simulink model "PUMA_8MM"  (Simulink 8.6)
settings: Solver=ode5  StartTime=0.0  StopTime=3  FixedStep=0.003  RelTol=1e-3
undefined symbols (not defined in the file): magnitude
libraries: vrlib x8, simulink x5
(part 1 of 2)
settings Model: Creator=Igor  LastModifiedBy=User
settings OptimizationCC: InitFltsAndDblsToZero=on
settings DebuggingCC: FcnCallInpInsideContextMsg=UseLocalSettings
settings SFSimCC: SimParseCustomCode=off

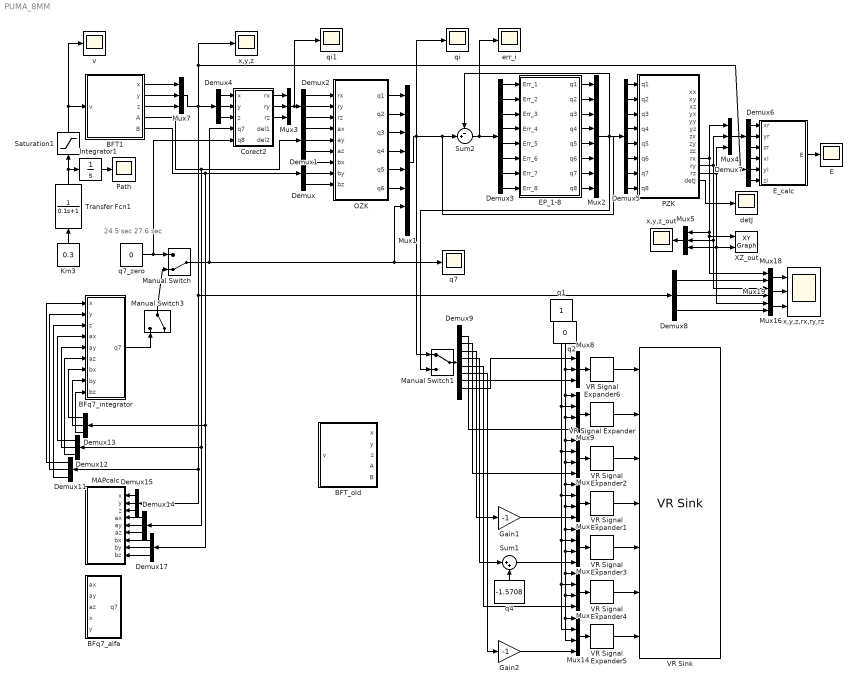
== system PUMA_8MM ==
  note: 24.5 sec
      | 27.6 sec
  BFT1 : Subsystem
  BFT_old : Subsystem
  BFq7_alfa : MATLAB Function  TreatAsAtomicUnit=on
  BFq7_integrator : Subsystem
  Corect2 : MATLAB Function  TreatAsAtomicUnit=on
  Demux{,1..2,4,6..8,11..15,17} (13 alike) : Demux  Outputs=3
  Demux3 : Demux  Outputs=8
  Demux5 : Demux  Outputs=8
  Demux9 : Demux  Outputs=8
  E : Scope
  EP_1-8 : Subsystem
  E_calc : MATLAB Function  TreatAsAtomicUnit=on
  Gain1 : Gain  Gain=-1
  Gain2 : Gain  Gain=-1
  Integrator1 : Integrator
  Km3 : Constant  Value=0.3
  MAPcalc : Subsystem
  Manual Switch : ManualSwitch  CurrentSetting=0
  Manual Switch1 : ManualSwitch
  Manual Switch3 : ManualSwitch  CurrentSetting=0
  Mux1 : Mux  Inputs=8
  Mux{9..14} (6 alike) : Mux
  Mux16 : Mux  Inputs=2
  Mux18 : Mux  Inputs=2
  Mux19 : Mux  Inputs=2
  Mux2 : Mux  Inputs=8
  Mux{3..5,7..8} (5 alike) : Mux  Inputs=3
  OZK : MATLAB Function  TreatAsAtomicUnit=on
  PZK : MATLAB Function  TreatAsAtomicUnit=on
  Path : Scope
  Saturation1 : Saturate  UpperLimit=10  LowerLimit=0.001
  Sum1 : Sum  Inputs=|++
  Sum2 : Sum  Inputs=-+|
  Transfer Fcn1 : TransferFcn  Denominator=[0.1 1]
  VR Signal Expander{,1..5} (6 alike) : vrlib/VR Signal Expander  outwidth=4  outidx=[1 2 3 4]
  VR Signal Expander6 : vrlib/VR Signal Expander  outwidth=3  outidx=[1 2 3]
  VR Sink : vrlib/VR Sink  InstantiateOnLoad=on  SampleTime=-1  ViewEnable=on  RemoteChange=off  RemoteView=off  FieldsWritten=q7_block1.translation.3.1.1.double#q1_block3.rotation.4.1.1.double#q2_block5.rotation.4.1.1.double#q3_block7.rotation.4.1.1.double#q4_block8.rotation.4.1.1.double#q5_block10.rotation.4.1.1.double#q6_block11.rotation.4.1.1.double  WorldFileName=MM_3Dmodel.wrl  WorldDescription=MM_3Dmodel  AutoView=on  VideoDimensions=[]  AllowVariableSize=off  FigureProperties="{'Position', 'Name', 'Viewpoint', 'CameraBound', 'CameraDirection', 'CameraPosition', 'CameraUpVector', 'ZoomFactor', 'Antialiasing', 'Headlight', 'Lighting', 'NavPanel', 'Sound', 'StatusBar', 'Stereo3D', 'Stereo3DCameraOffset', 'Stereo3DHIT', 'ToolBar', 'Textures', 'Transparency', 'Triad', 'Wireframe', 'NavZones', 'NavMode', 'NavSpeed', 'CaptureFileFormat', 'CaptureFileName', 'Record2DCompressMethod', 'Record2DCompressQuality', 'Record2D', 'Record2DFileName', 'Record2DFPS'; [9.3400000000000000e+02   2.7200000000000000e+02   8.2600000000000000e+02   5.2800000000000000e+02], 'MM_3Dmodel', '', 'on', [-6.5943356188839664e-01  -2.5114047294941466e-01  -7.0857310159359332e-01], [2.3358426713746256e+00   1.1531799680057284e+00   2.3142922974527869e+00], [-1.9468492056750838e-01   9.6744405949295276e-01  -1.6170891581923202e-01], [1.0000000000000000e+00], 'on', 'on', 'on', 'halfbar', 'on', 'on', 'off', [1.0000000149011612e-01], [0.0000000000000000e+00], 'on', 'on', 'on', 'none', 'off', 'off', 'fly', 'normal', 'tif', '%f_anim_%n.tif', 'auto', [7.5000000000000000e+01], 'off', '%f_anim_%n.avi', [1.5000000000000000e+01]}"
  XZ_out : simulink/Sinks/XY Graph  xmin=-0.5  xmax=1.5  ymin=-0.5  ymax=1.5  st=-1
  detJ : Scope
  err_i : Scope
  q1 : Constant
  q2 : Constant  Value=0
  q4 : Constant  Value=-1.5708
  q7 : Scope
  q7_zero : Constant  Value=0
  qi : Scope
  qi1 : Scope
  v : Scope
  x,y,z : Scope
  x,y,z,rx,ry,rz : Scope  NumInputPorts=3
  x,y,z_out : Scope
  wires:
  E_calc/1(E) -> E/1
  Integrator1/1 -> Path/1
  Saturation1/1 -> v/1, BFT1/1(v)
  Demux/1 -> OZK/7(bx)
  Demux/2 -> OZK/8(by)
  Demux/3 -> OZK/9(bz)
  Demux1/1 -> OZK/4(ax)
  Demux1/2 -> OZK/5(ay)
  Demux1/3 -> OZK/6(az)
  Demux2/1 -> OZK/1(rx)
  Demux2/2 -> OZK/2(ry)
  Demux2/3 -> OZK/3(rz)
  Mux1/1 -> Sum2/2, Demux5/1, Manual Switch1/1, qi/1
  BFT1/3(z) -> Mux7/3
  Demux3/1 -> EP_1-8/1(Err_1)
  Demux3/2 -> EP_1-8/2(Err_2)
  Demux3/3 -> EP_1-8/3(Err_3)
  Demux3/4 -> EP_1-8/4(Err_4)
  Demux3/5 -> EP_1-8/5(Err_5)
  Demux3/6 -> EP_1-8/6(Err_6)
  EP_1-8/1(q1) -> Mux2/1
  EP_1-8/2(q2) -> Mux2/2
  EP_1-8/3(q3) -> Mux2/3
  EP_1-8/4(q4) -> Mux2/4
  EP_1-8/5(q5) -> Mux2/5
  EP_1-8/6(q6) -> Mux2/6
  Demux3/7 -> EP_1-8/7(Err_7)
  Demux3/8 -> EP_1-8/8(Err_8)
  EP_1-8/7(q7) -> Mux2/7
  EP_1-8/8(q8) -> Mux2/8
  Mux7/1 -> Demux4/1, Demux8/1, Demux11/1, Demux15/1, Demux7/1, x,y,z/1
  Demux5/1 -> PZK/1(q1)
  Demux5/2 -> PZK/2(q2)
  Demux5/3 -> PZK/3(q3)
  Demux5/4 -> PZK/4(q4)
  Demux5/5 -> PZK/5(q5)
  Demux5/6 -> PZK/6(q6)
  Demux5/7 -> PZK/7(q7)
  Demux5/8 -> PZK/8(q8)
  Demux6/1 -> E_calc/1(xr)
  Demux6/2 -> E_calc/2(yr)
  Demux6/3 -> E_calc/3(zr)
  Mux4/1 -> Demux6/1
  Demux7/1 -> E_calc/4(xi)
  Demux7/2 -> E_calc/5(yi)
  Demux7/3 -> E_calc/6(zi)
  OZK/1(q1) -> Mux1/1
  OZK/3(q3) -> Mux1/3
  OZK/2(q2) -> Mux1/2
  OZK/4(q4) -> Mux1/4
  OZK/5(q5) -> Mux1/5
  OZK/6(q6) -> Mux1/6
  Demux8/3 -> Mux16/2
  Demux8/2 -> Mux19/2
  Demux8/1 -> Mux18/2
  Mux18/1 -> x,y,z,rx,ry,rz/1
  Mux19/1 -> x,y,z,rx,ry,rz/2
  Mux16/1 -> x,y,z,rx,ry,rz/3
  PZK/10(rx) -> Mux4/1, Mux18/1, XZ_out/1, Mux5/1
  PZK/11(ry) -> Mux4/2, Mux5/2, Mux19/1
  PZK/12(rz) -> Mux4/3, Mux16/1, XZ_out/2, Mux5/3
  Mux3/1 -> qi1/1, Demux2/1
  Mux8/1 -> VR Signal Expander6/1
  q2/1 -> Mux8/2, Mux9/1, Mux9/3, Mux11/1, Mux10/1, Mux10/3, Mux12/1, Mux12/3, Mux13/1, Mux13/3, Mux14/1, Mux14/3, Mux11/3
  Mux9/1 -> VR Signal Expander/1
  q1/1 -> Mux9/2, Mux11/2, Mux10/2, Mux12/2, Mux13/2, Mux14/2
  Demux9/1 -> Mux9/4
  Demux9/7 -> Mux8/3
  Mux10/1 -> VR Signal Expander1/1
  Demux9/3 -> Gain1/1
  Mux11/1 -> VR Signal Expander2/1
  Demux9/2 -> Mux11/4
  Mux12/1 -> VR Signal Expander3/1
  Demux9/4 -> Sum1/1
  Mux13/1 -> VR Signal Expander4/1
  Demux9/5 -> Mux13/4
  Demux9/8 -> Mux8/1
  Mux14/1 -> VR Signal Expander5/1
  Gain1/1 -> Mux10/4
  Demux9/6 -> Gain2/1
  VR Signal Expander6/1 -> VR Sink/1
  VR Signal Expander/1 -> VR Sink/2
  VR Signal Expander2/1 -> VR Sink/3
  VR Signal Expander1/1 -> VR Sink/4
  VR Signal Expander3/1 -> VR Sink/5
  VR Signal Expander4/1 -> VR Sink/6
  VR Signal Expander5/1 -> VR Sink/7
  Gain2/1 -> Mux14/4
  Manual Switch1/1 -> Demux9/1
  Sum1/1 -> Mux12/4
  q4/1 -> Sum1/2
  Sum2/1 -> err_i/1, Demux3/1
  q7_zero/1 -> Manual Switch/1, Corect2/5(q8)
  BFT1/2(y) -> Mux7/2
  BFT1/1(x) -> Mux7/1
  BFT1/4(A) -> Demux12/1, Demux14/1, Demux1/1
  BFT1/5(B) -> Demux13/1, Demux17/1, Demux/1
  Mux2/1 -> Manual Switch1/2, Sum2/1
  Demux11/1 -> BFq7_integrator/1(x)
  Demux11/2 -> BFq7_integrator/2(y)
  Demux11/3 -> BFq7_integrator/3(z)
  Demux12/1 -> BFq7_integrator/4(ax)
  Demux12/2 -> BFq7_integrator/5(ay)
  Demux12/3 -> BFq7_integrator/6(az)
  Demux13/1 -> BFq7_integrator/7(bx)
  Demux13/2 -> BFq7_integrator/8(by)
  Demux13/3 -> BFq7_integrator/9(bz)
  Manual Switch3/1 -> Manual Switch/2
  BFq7_integrator/1(q7) -> Manual Switch3/1
  Km3/1 -> Transfer Fcn1/1
  Transfer Fcn1/1 -> Saturation1/1, Integrator1/1
  PZK/13(detJ) -> detJ/1
  Demux17/3 -> MAPcalc/9(bz)
  Demux17/2 -> MAPcalc/8(by)
  Demux17/1 -> MAPcalc/7(bx)
  Demux14/3 -> MAPcalc/6(az)
  Demux14/2 -> MAPcalc/5(ay)
  Demux14/1 -> MAPcalc/4(ax)
  Demux15/3 -> MAPcalc/3(z)
  Demux15/2 -> MAPcalc/2(y)
  Demux15/1 -> MAPcalc/1(x)
  Manual Switch/1 -> q7/1, Mux1/7, Corect2/4(q7)
  Corect2/1(rx) -> Mux3/1
  Corect2/2(ry) -> Mux3/2
  Corect2/3(rz) -> Mux3/3
  Demux4/1 -> Corect2/1(x)
  Demux4/2 -> Corect2/2(y)
  Demux4/3 -> Corect2/3(z)
  Mux5/1 -> x,y,z_out/1

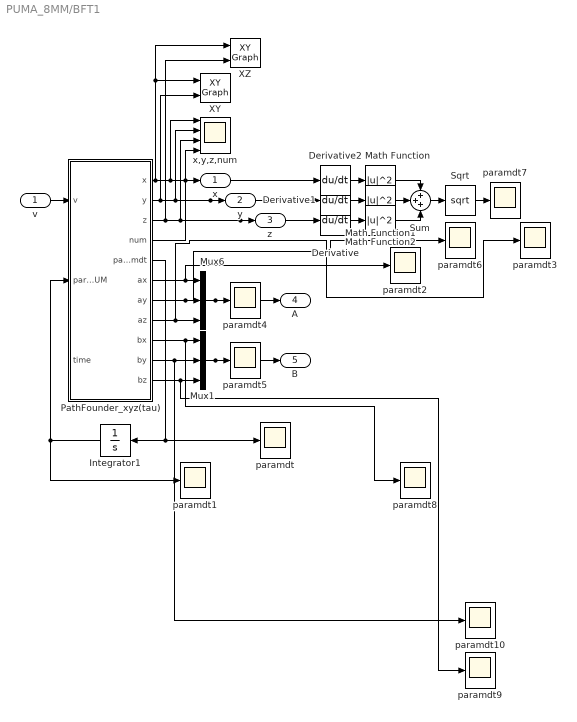
== system PUMA_8MM/BFT1 ==
  v : Inport
  Derivative : Derivative
  Derivative1 : Derivative
  Derivative2 : Derivative
  Integrator1 : Integrator
  Math Function : Math  Operator=magnitude^2  SaturateOnIntegerOverflow=on
  Math Function1 : Math  Operator=magnitude^2  SaturateOnIntegerOverflow=on
  Math Function2 : Math  Operator=magnitude^2  SaturateOnIntegerOverflow=on
  Mux1 : Mux  Inputs=3
  Mux6 : Mux  Inputs=3
  PathFounder_xyz(tau) : MATLAB Function  TreatAsAtomicUnit=on
  Sqrt : Sqrt  SaturateOnIntegerOverflow=on
  Sum : Sum  Inputs=+++
  XY : simulink/Sinks/XY Graph  xmin=-0.5  xmax=1.5  ymin=0  ymax=2  st=-1
  XZ : simulink/Sinks/XY Graph  xmin=-0.5  xmax=1.5  ymin=-0.5  ymax=1.5  st=-1
  paramdt{,1..10} (11 alike) : Scope
  x,y,z,num : Scope  NumInputPorts=4
  x : Outport
  y : Outport  Port=2
  z : Outport  Port=3
  A : Outport  Port=4
  B : Outport  Port=5
  wires:
  v/1 -> PathFounder_xyz(tau)/1(v)
  PathFounder_xyz(tau)/4(num) -> x,y,z,num/4
  PathFounder_xyz(tau)/3(z) -> XZ/2, z/1, Derivative/1, x,y,z,num/3
  PathFounder_xyz(tau)/2(y) -> y/1, Derivative1/1, x,y,z,num/2, XY/2
  PathFounder_xyz(tau)/1(x) -> x/1, Derivative2/1, x,y,z,num/1, XY/1, XZ/1
  Integrator1/1 -> paramdt1/1, PathFounder_xyz(tau)/2(paramSUM)
  PathFounder_xyz(tau)/5(paramdt) -> Integrator1/1, paramdt/1
  Mux6/1 -> paramdt4/1, A/1
  Mux1/1 -> paramdt5/1, B/1
  Derivative/1 -> Math Function2/1
  Derivative1/1 -> Math Function1/1
  Derivative2/1 -> Math Function/1
  Math Function2/1 -> Sum/3
  Math Function1/1 -> Sum/2
  Math Function/1 -> Sum/1
  Sum/1 -> Sqrt/1
  Sqrt/1 -> paramdt7/1
  PathFounder_xyz(tau)/6(ax) -> paramdt2/1, Mux6/1
  PathFounder_xyz(tau)/7(ay) -> paramdt6/1, Mux6/2
  PathFounder_xyz(tau)/8(az) -> Mux6/3, paramdt3/1
  PathFounder_xyz(tau)/9(bx) -> paramdt8/1, Mux1/1
  PathFounder_xyz(tau)/10(by) -> paramdt10/1, Mux1/2
  PathFounder_xyz(tau)/11(bz) -> paramdt9/1, Mux1/3

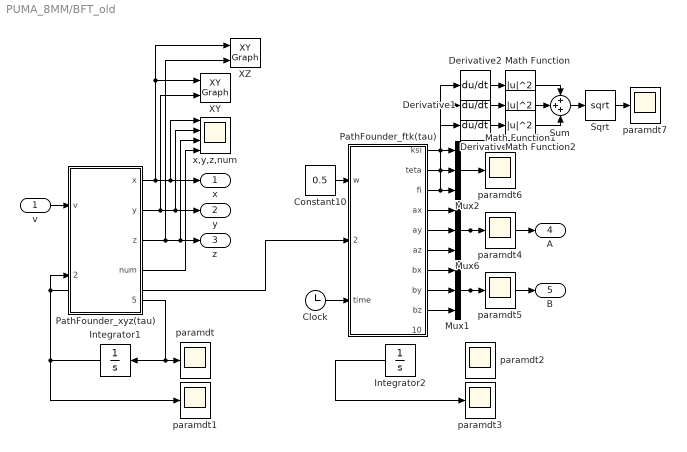
== system PUMA_8MM/BFT_old ==
  v : Inport
  Clock : Clock
  Constant10 : Constant  Value=0.5
  Derivative : Derivative
  Derivative1 : Derivative
  Derivative2 : Derivative
  Integrator1 : Integrator
  Integrator2 : Integrator
  Math Function : Math  Operator=magnitude^2  SaturateOnIntegerOverflow=on
  Math Function1 : Math  Operator=magnitude^2  SaturateOnIntegerOverflow=on
  Math Function2 : Math  Operator=magnitude^2  SaturateOnIntegerOverflow=on
  Mux1 : Mux  Inputs=3
  Mux2 : Mux  Inputs=3
  Mux6 : Mux  Inputs=3
  PathFounder_ftk(tau) : MATLAB Function  TreatAsAtomicUnit=on
  PathFounder_xyz(tau) : MATLAB Function  TreatAsAtomicUnit=on
  Sqrt : Sqrt  SaturateOnIntegerOverflow=on
  Sum : Sum  Inputs=+++
  XY : simulink/Sinks/XY Graph  xmin=-1  xmax=1  ymin=0  ymax=2  st=-1
  XZ : simulink/Sinks/XY Graph  xmin=-0.5  xmax=0.5  ymin=-0.4  ymax=1  st=-1
  paramdt{,1..7} (8 alike) : Scope
  x,y,z,num : Scope  NumInputPorts=4
  x : Outport
  y : Outport  Port=2
  z : Outport  Port=3
  A : Outport  Port=4
  B : Outport  Port=5
  wires:
  v/1 -> PathFounder_xyz(tau)/1(v)
  PathFounder_xyz(tau)/4(num) -> x,y,z,num/4
  PathFounder_xyz(tau)/3(z) -> x,y,z,num/3, z/1, XZ/2
  PathFounder_xyz(tau)/2(y) -> x,y,z,num/2, y/1, XY/2
  PathFounder_xyz(tau)/1(x) -> x,y,z,num/1, x/1, XY/1, XZ/1
  Integrator1/1 -> paramdt1/1, PathFounder_xyz(tau)/2(paramSUM), PathFounder_ftk(tau)/2(paramSUM)
  PathFounder_xyz(tau)/5(paramdt) -> Integrator1/1, paramdt/1
  Integrator2/1 -> paramdt3/1
  Constant10/1 -> PathFounder_ftk(tau)/1(w)
  PathFounder_ftk(tau)/4(ax) -> Mux6/1
  PathFounder_ftk(tau)/5(ay) -> Mux6/2
  PathFounder_ftk(tau)/6(az) -> Mux6/3
  PathFounder_ftk(tau)/7(bx) -> Mux1/1
  PathFounder_ftk(tau)/8(by) -> Mux1/2
  PathFounder_ftk(tau)/9(bz) -> Mux1/3
  Mux6/1 -> paramdt4/1, A/1
  Mux1/1 -> paramdt5/1, B/1
  Mux2/1 -> paramdt6/1
  PathFounder_ftk(tau)/3(fi) -> Mux2/3, Derivative/1
  PathFounder_ftk(tau)/2(teta) -> Mux2/2, Derivative1/1
  PathFounder_ftk(tau)/1(ksi) -> Mux2/1, Derivative2/1
  Derivative/1 -> Math Function2/1
  Derivative1/1 -> Math Function1/1
  Derivative2/1 -> Math Function/1
  Math Function2/1 -> Sum/3
  Math Function1/1 -> Sum/2
  Math Function/1 -> Sum/1
  Sum/1 -> Sqrt/1
  Sqrt/1 -> paramdt7/1
  Clock/1 -> PathFounder_ftk(tau)/3(time)

== system PUMA_8MM/BFq7_integrator ==
  x : Inport
  y : Inport  Port=2
  z : Inport  Port=3
  ax : Inport  Port=4
  ay : Inport  Port=5
  az : Inport  Port=6
  bx : Inport  Port=7
  by : Inport  Port=8
  bz : Inport  Port=9
  Integrator1 : Integrator
  Mux7 : Mux  Inputs=3
  OZK_q7+ : MATLAB Function  TreatAsAtomicUnit=on
  Path1 : Scope
  Path2 : Scope
  q7 : Outport
  wires:
  bx/1 -> OZK_q7+/7(bx)
  by/1 -> OZK_q7+/8(by)
  bz/1 -> OZK_q7+/9(bz)
  ax/1 -> OZK_q7+/4(ax)
  ay/1 -> OZK_q7+/5(ay)
  az/1 -> OZK_q7+/6(az)
  OZK_q7+/1(q7pr) -> Integrator1/1
  Integrator1/1 -> q7/1, OZK_q7+/10(q7)
  x/1 -> OZK_q7+/1(x)
  y/1 -> OZK_q7+/2(y)
  z/1 -> OZK_q7+/3(z)
  Mux7/1 -> Path1/1
  OZK_q7+/3(o2) -> Mux7/2
  OZK_q7+/2(o1) -> Mux7/1, Path2/1
  OZK_q7+/4(o3) -> Mux7/3

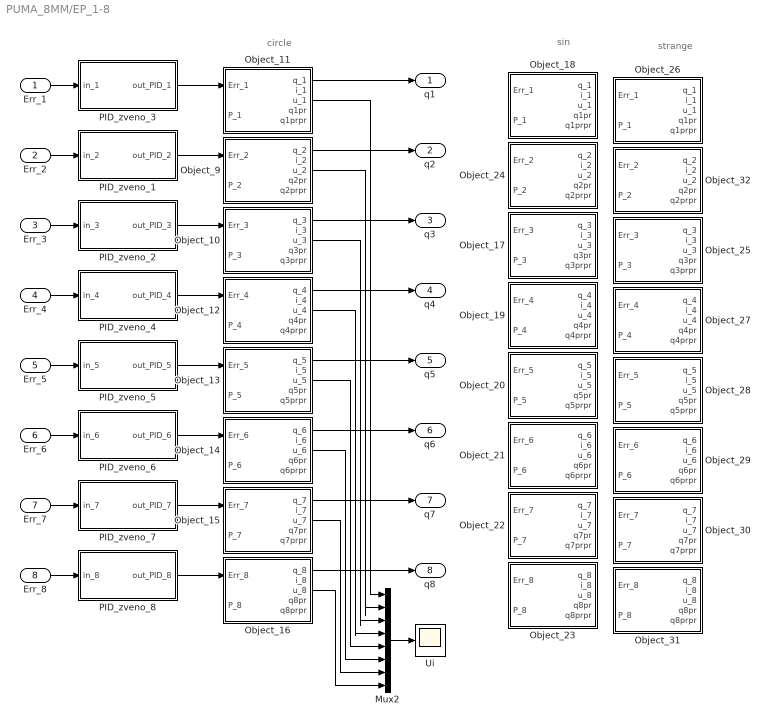
== system PUMA_8MM/EP_1-8 ==
  note: strange
  note: circle
  note: sin
  Err_1 : Inport
  Err_2 : Inport  Port=2
  Err_3 : Inport  Port=3
  Err_4 : Inport  Port=4
  Err_5 : Inport  Port=5
  Err_6 : Inport  Port=6
  Err_7 : Inport  Port=7
  Err_8 : Inport  Port=8
  Mux2 : Mux  Inputs=8
  Object_10 : Subsystem
  Object_11 : Subsystem
  Object_12 : Subsystem
  Object_13 : Subsystem
  Object_14 : Subsystem
  Object_15 : Subsystem
  Object_16 : Subsystem
  Object_17 : Subsystem
  Object_18 : Subsystem
  Object_19 : Subsystem
  Object_20 : Subsystem
  Object_21 : Subsystem
  Object_22 : Subsystem
  Object_23 : Subsystem
  Object_24 : Subsystem
  Object_25 : Subsystem
  Object_26 : Subsystem
  Object_27 : Subsystem
  Object_28 : Subsystem
  Object_29 : Subsystem
  Object_30 : Subsystem
  Object_31 : Subsystem
  Object_32 : Subsystem
  Object_9 : Subsystem
  PID_zveno_1 : Subsystem
  PID_zveno_2 : Subsystem
  PID_zveno_3 : Subsystem
  PID_zveno_4 : Subsystem
  PID_zveno_5 : Subsystem
  PID_zveno_6 : Subsystem
  PID_zveno_7 : Subsystem
  PID_zveno_8 : Subsystem
  Ui : Scope
  q1 : Outport
  q2 : Outport  Port=2
  q3 : Outport  Port=3
  q4 : Outport  Port=4
  q5 : Outport  Port=5
  q6 : Outport  Port=6
  q7 : Outport  Port=7
  q8 : Outport  Port=8
  wires:
  PID_zveno_3/1(out_PID_1) -> Object_11/1(Err_1)
  Err_1/1 -> PID_zveno_3/1(in_1)
  PID_zveno_1/1(out_PID_2) -> Object_9/1(Err_2)
  Err_2/1 -> PID_zveno_1/1(in_2)
  PID_zveno_2/1(out_PID_3) -> Object_10/1(Err_3)
  Err_3/1 -> PID_zveno_2/1(in_3)
  PID_zveno_4/1(out_PID_4) -> Object_12/1(Err_4)
  PID_zveno_5/1(out_PID_5) -> Object_13/1(Err_5)
  PID_zveno_6/1(out_PID_6) -> Object_14/1(Err_6)
  Err_4/1 -> PID_zveno_4/1(in_4)
  Err_5/1 -> PID_zveno_5/1(in_5)
  Err_6/1 -> PID_zveno_6/1(in_6)
  PID_zveno_7/1(out_PID_7) -> Object_15/1(Err_7)
  Err_7/1 -> PID_zveno_7/1(in_7)
  PID_zveno_8/1(out_PID_8) -> Object_16/1(Err_8)
  Err_8/1 -> PID_zveno_8/1(in_8)
  Object_11/1(q_1) -> q1/1
  Object_9/1(q_2) -> q2/1
  Object_15/1(q_7) -> q7/1
  Object_16/1(q_8) -> q8/1
  Object_14/1(q_6) -> q6/1
  Object_13/1(q_5) -> q5/1
  Object_12/1(q_4) -> q4/1
  Object_10/1(q_3) -> q3/1
  Mux2/1 -> Ui/1
  Object_11/3(u_1) -> Mux2/1
  Object_9/3(u_2) -> Mux2/2
  Object_10/3(u_3) -> Mux2/3
  Object_12/3(u_4) -> Mux2/4
  Object_13/3(u_5) -> Mux2/5
  Object_14/3(u_6) -> Mux2/6
  Object_15/3(u_7) -> Mux2/7
  Object_16/3(u_8) -> Mux2/8

== system PUMA_8MM/MAPcalc ==
  note: Y = [-0.95 -0.9 -0.85 -0.8 -0.75 -0.7 -0.65 -0.6 -0.55 -0.5 -0.45 -0.4 -0.35 -0.3 -0.25 -0.2 -0.15 -0.1 -0.05 0 0.05 0.1 0.15 0.2 0.25 0.3 0.35 0.4 0.45 0.5 0.55 0.6 0.65 0.7 0.75 0.8 0.85 0.9 0.95];
  note: mesh(Y,MAP.time,MAP.signals.values)
  note: Y = [0.95 0.9 0.85 0.8 0.75 0.7 0.65 0.6 0.55 0.5 0.45 0.4 0.35 0.3 0.25 0.2 0.15 0.1 0.05 0 -0.05 -0.1 -0.15 -0.2 -0.25 -0.3 -0.35 -0.4 -0.45 -0.5 -0.55 -0.6 -0.65 -0.7 -0.75 -0.8 -0.85 -0.9 -0.95];
  x : Inport
  y : Inport  Port=2
  z : Inport  Port=3
  ax : Inport  Port=4
  ay : Inport  Port=5
  az : Inport  Port=6
  bx : Inport  Port=7
  by : Inport  Port=8
  bz : Inport  Port=9
  MAP : Scope
  Mux3 : Mux  Inputs=39
  OZK_q7+ : MATLAB Function  TreatAsAtomicUnit=on
  Saturation1 : Saturate  UpperLimit=1  LowerLimit=0
  wires:
  z/1 -> OZK_q7+/3(z)
  y/1 -> OZK_q7+/2(y)
  x/1 -> OZK_q7+/1(x)
  az/1 -> OZK_q7+/6(az)
  ay/1 -> OZK_q7+/5(ay)
  ax/1 -> OZK_q7+/4(ax)
  bz/1 -> OZK_q7+/9(bz)
  by/1 -> OZK_q7+/8(by)
  bx/1 -> OZK_q7+/7(bx)
  Mux3/1 -> Saturation1/1
  Saturation1/1 -> MAP/1
  OZK_q7+/39(M40) -> Mux3/39
  OZK_q7+/38(M39) -> Mux3/38
  OZK_q7+/37(M38) -> Mux3/37
  OZK_q7+/36(M37) -> Mux3/36
  OZK_q7+/35(M36) -> Mux3/35
  OZK_q7+/34(M35) -> Mux3/34
  OZK_q7+/33(M34) -> Mux3/33
  OZK_q7+/32(M33) -> Mux3/32
  OZK_q7+/31(M32) -> Mux3/31
  OZK_q7+/30(M31) -> Mux3/30
  OZK_q7+/29(M30) -> Mux3/29
  OZK_q7+/28(M29) -> Mux3/28
  OZK_q7+/27(M28) -> Mux3/27
  OZK_q7+/26(M27) -> Mux3/26
  OZK_q7+/25(M26) -> Mux3/25
  OZK_q7+/24(M25) -> Mux3/24
  OZK_q7+/23(M24) -> Mux3/23
  OZK_q7+/22(M23) -> Mux3/22
  OZK_q7+/21(M22) -> Mux3/21
  OZK_q7+/20(M21) -> Mux3/20
  OZK_q7+/19(M20) -> Mux3/19
  OZK_q7+/18(M19) -> Mux3/18
  OZK_q7+/16(M17) -> Mux3/16
  OZK_q7+/17(M18) -> Mux3/17
  OZK_q7+/15(M16) -> Mux3/15
  OZK_q7+/14(M15) -> Mux3/14
  OZK_q7+/13(M14) -> Mux3/13
  OZK_q7+/12(M13) -> Mux3/12
  OZK_q7+/11(M12) -> Mux3/11
  OZK_q7+/10(M11) -> Mux3/10
  OZK_q7+/9(M10) -> Mux3/9
  OZK_q7+/8(M9) -> Mux3/8
  OZK_q7+/7(M8) -> Mux3/7
  OZK_q7+/6(M7) -> Mux3/6
  OZK_q7+/5(M6) -> Mux3/5
  OZK_q7+/4(M5) -> Mux3/4
  OZK_q7+/3(M4) -> Mux3/3
  OZK_q7+/2(M3) -> Mux3/2
  OZK_q7+/1(M2) -> Mux3/1

== system PUMA_8MM/EP_1-8/Object_10 ==
  Err_3 : Inport
  P_3 : Inport  Port=2
  Gain1 : Gain  Gain=0.04
  Gain{2..3,6..7} (4 alike) : Gain  Gain=1/102.5
  Gain4 : Gain  Gain=1/(3.5*0.0001)
  Gain5 : Gain  Gain=0.04
  Integrator1 : Integrator
  Integrator7 : Integrator  InitialCondition=-1.3925*102.5
  Sum1 : Sum  Inputs=|+-
  Sum2 : Sum  Inputs=|+-
  Transfer Fcn2 : TransferFcn  Denominator=[0.0075 0.5]
  q_3 : Outport
  i_3 : Outport  Port=2
  u_3 : Outport  Port=3
  q3pr : Outport  Port=4
  q3prpr : Outport  Port=5
  wires:
  Gain7/1 -> q3prpr/1
  Gain3/1 -> q3pr/1
  Gain2/1 -> Sum2/2
  Gain6/1 -> q_3/1
  P_3/1 -> Gain2/1
  Err_3/1 -> u_3/1, Sum1/1
  Sum2/1 -> Gain4/1
  Gain4/1 -> Gain7/1, Integrator1/1
  Sum1/1 -> Transfer Fcn2/1
  Gain5/1 -> Sum1/2
  Integrator7/1 -> Gain6/1
  Integrator1/1 -> Integrator7/1, Gain3/1, Gain5/1
  Gain1/1 -> Sum2/1
  Transfer Fcn2/1 -> Gain1/1, i_3/1

== system PUMA_8MM/EP_1-8/Object_11 ==
  Err_1 : Inport
  P_1 : Inport  Port=2
  Gain1 : Gain  Gain=0.04
  Gain{2..3,6..7} (4 alike) : Gain  Gain=1/102.5
  Gain4 : Gain  Gain=1/(3.5*0.0001)
  Gain5 : Gain  Gain=0.04
  Integrator1 : Integrator
  Integrator7 : Integrator  InitialCondition=0*102.5
  Sum1 : Sum  Inputs=|+-
  Sum2 : Sum  Inputs=|+-
  Transfer Fcn2 : TransferFcn  Denominator=[0.0075 0.5]
  q_1 : Outport
  i_1 : Outport  Port=2
  u_1 : Outport  Port=3
  q1pr : Outport  Port=4
  q1prpr : Outport  Port=5
  wires:
  Gain7/1 -> q1prpr/1
  Gain3/1 -> q1pr/1
  Gain2/1 -> Sum2/2
  Gain6/1 -> q_1/1
  P_1/1 -> Gain2/1
  Err_1/1 -> u_1/1, Sum1/1
  Sum2/1 -> Gain4/1
  Gain4/1 -> Gain7/1, Integrator1/1
  Sum1/1 -> Transfer Fcn2/1
  Gain5/1 -> Sum1/2
  Integrator7/1 -> Gain6/1
  Integrator1/1 -> Integrator7/1, Gain3/1, Gain5/1
  Gain1/1 -> Sum2/1
  Transfer Fcn2/1 -> Gain1/1, i_1/1

== system PUMA_8MM/EP_1-8/Object_12 ==
  Err_4 : Inport
  P_4 : Inport  Port=2
  Gain1 : Gain  Gain=0.04
  Gain{2..3,6..7} (4 alike) : Gain  Gain=1/102.5
  Gain4 : Gain  Gain=1/(3.5*0.0001)
  Gain5 : Gain  Gain=0.04
  Integrator1 : Integrator
  Integrator7 : Integrator  InitialCondition=1.57*102.5
  Sum1 : Sum  Inputs=|+-
  Sum2 : Sum  Inputs=|+-
  Transfer Fcn2 : TransferFcn  Denominator=[0.0075 0.5]
  q_4 : Outport
  i_4 : Outport  Port=2
  u_4 : Outport  Port=3
  q4pr : Outport  Port=4
  q4prpr : Outport  Port=5
  wires:
  Transfer Fcn2/1 -> i_4/1, Gain1/1
  Gain1/1 -> Sum2/1
  Integrator1/1 -> Gain5/1, Gain3/1, Integrator7/1
  Integrator7/1 -> Gain6/1
  Gain5/1 -> Sum1/2
  Sum1/1 -> Transfer Fcn2/1
  Gain4/1 -> Integrator1/1, Gain7/1
  Sum2/1 -> Gain4/1
  Err_4/1 -> Sum1/1, u_4/1
  P_4/1 -> Gain2/1
  Gain6/1 -> q_4/1
  Gain2/1 -> Sum2/2
  Gain3/1 -> q4pr/1
  Gain7/1 -> q4prpr/1

== system PUMA_8MM/EP_1-8/Object_13 ==
  Err_5 : Inport
  P_5 : Inport  Port=2
  Gain1 : Gain  Gain=0.04
  Gain{2..3,6..7} (4 alike) : Gain  Gain=1/102.5
  Gain4 : Gain  Gain=1/(3.5*0.0001)
  Gain5 : Gain  Gain=0.04
  Integrator1 : Integrator
  Integrator7 : Integrator  InitialCondition=0.603*102.5
  Sum1 : Sum  Inputs=|+-
  Sum2 : Sum  Inputs=|+-
  Transfer Fcn2 : TransferFcn  Denominator=[0.0075 0.5]
  q_5 : Outport
  i_5 : Outport  Port=2
  u_5 : Outport  Port=3
  q5pr : Outport  Port=4
  q5prpr : Outport  Port=5
  wires:
  Gain7/1 -> q5prpr/1
  Gain3/1 -> q5pr/1
  Gain2/1 -> Sum2/2
  Gain6/1 -> q_5/1
  P_5/1 -> Gain2/1
  Err_5/1 -> u_5/1, Sum1/1
  Sum2/1 -> Gain4/1
  Gain4/1 -> Gain7/1, Integrator1/1
  Sum1/1 -> Transfer Fcn2/1
  Gain5/1 -> Sum1/2
  Integrator7/1 -> Gain6/1
  Integrator1/1 -> Integrator7/1, Gain3/1, Gain5/1
  Gain1/1 -> Sum2/1
  Transfer Fcn2/1 -> Gain1/1, i_5/1

== system PUMA_8MM/EP_1-8/Object_14 ==
  Err_6 : Inport
  P_6 : Inport  Port=2
  Gain1 : Gain  Gain=0.04
  Gain{2..3,6..7} (4 alike) : Gain  Gain=1/102.5
  Gain4 : Gain  Gain=1/(3.5*0.0001)
  Gain5 : Gain  Gain=0.04
  Integrator1 : Integrator
  Integrator7 : Integrator  InitialCondition=-1.57*102.5
  Sum1 : Sum  Inputs=|+-
  Sum2 : Sum  Inputs=|+-
  Transfer Fcn2 : TransferFcn  Denominator=[0.0075 0.5]
  q_6 : Outport
  i_6 : Outport  Port=2
  u_6 : Outport  Port=3
  q6pr : Outport  Port=4
  q6prpr : Outport  Port=5
  wires:
  Transfer Fcn2/1 -> i_6/1, Gain1/1
  Gain1/1 -> Sum2/1
  Integrator1/1 -> Gain5/1, Gain3/1, Integrator7/1
  Integrator7/1 -> Gain6/1
  Gain5/1 -> Sum1/2
  Sum1/1 -> Transfer Fcn2/1
  Gain4/1 -> Integrator1/1, Gain7/1
  Sum2/1 -> Gain4/1
  Err_6/1 -> Sum1/1, u_6/1
  P_6/1 -> Gain2/1
  Gain6/1 -> q_6/1
  Gain2/1 -> Sum2/2
  Gain3/1 -> q6pr/1
  Gain7/1 -> q6prpr/1

== system PUMA_8MM/EP_1-8/Object_15 ==
  Err_7 : Inport
  P_7 : Inport  Port=2
  Gain1 : Gain  Gain=0.04
  Gain{2..3,6..7} (4 alike) : Gain  Gain=1/102.5
  Gain4 : Gain  Gain=1/(3.5*0.0001)
  Gain5 : Gain  Gain=0.04
  Integrator1 : Integrator
  Integrator7 : Integrator  InitialCondition=0.35*102.5
  Sum1 : Sum  Inputs=|+-
  Sum2 : Sum  Inputs=|+-
  Transfer Fcn2 : TransferFcn  Denominator=[0.0075 0.5]
  q_7 : Outport
  i_7 : Outport  Port=2
  u_7 : Outport  Port=3
  q7pr : Outport  Port=4
  q7prpr : Outport  Port=5
  wires:
  Gain7/1 -> q7prpr/1
  Gain3/1 -> q7pr/1
  Gain2/1 -> Sum2/2
  Gain6/1 -> q_7/1
  P_7/1 -> Gain2/1
  Err_7/1 -> u_7/1, Sum1/1
  Sum2/1 -> Gain4/1
  Gain4/1 -> Gain7/1, Integrator1/1
  Sum1/1 -> Transfer Fcn2/1
  Gain5/1 -> Sum1/2
  Integrator7/1 -> Gain6/1
  Integrator1/1 -> Integrator7/1, Gain3/1, Gain5/1
  Gain1/1 -> Sum2/1
  Transfer Fcn2/1 -> Gain1/1, i_7/1

== system PUMA_8MM/EP_1-8/Object_16 ==
  Err_8 : Inport
  P_8 : Inport  Port=2
  Gain1 : Gain  Gain=0.04
  Gain{2..3,6..7} (4 alike) : Gain  Gain=1/102.5
  Gain4 : Gain  Gain=1/(3.5*0.0001)
  Gain5 : Gain  Gain=0.04
  Integrator1 : Integrator
  Integrator7 : Integrator  InitialCondition=0*102.5
  Sum1 : Sum  Inputs=|+-
  Sum2 : Sum  Inputs=|+-
  Transfer Fcn2 : TransferFcn  Denominator=[0.0075 0.5]
  q_8 : Outport
  i_8 : Outport  Port=2
  u_8 : Outport  Port=3
  q8pr : Outport  Port=4
  q8prpr : Outport  Port=5
  wires:
  Transfer Fcn2/1 -> i_8/1, Gain1/1
  Gain1/1 -> Sum2/1
  Integrator1/1 -> Gain5/1, Gain3/1, Integrator7/1
  Integrator7/1 -> Gain6/1
  Gain5/1 -> Sum1/2
  Sum1/1 -> Transfer Fcn2/1
  Gain4/1 -> Integrator1/1, Gain7/1
  Sum2/1 -> Gain4/1
  Err_8/1 -> Sum1/1, u_8/1
  P_8/1 -> Gain2/1
  Gain6/1 -> q_8/1
  Gain2/1 -> Sum2/2
  Gain3/1 -> q8pr/1
  Gain7/1 -> q8prpr/1

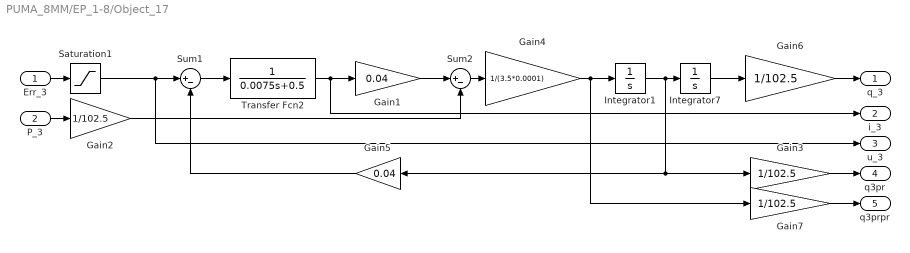
== system PUMA_8MM/EP_1-8/Object_17 ==
  Err_3 : Inport
  P_3 : Inport  Port=2
  Gain1 : Gain  Gain=0.04
  Gain{2..3,6..7} (4 alike) : Gain  Gain=1/102.5
  Gain4 : Gain  Gain=1/(3.5*0.0001)
  Gain5 : Gain  Gain=0.04
  Integrator1 : Integrator
  Integrator7 : Integrator  InitialCondition=-1.3338*102.5
  Saturation1 : Saturate  UpperLimit=30  LowerLimit=-30
  Sum1 : Sum  Inputs=|+-
  Sum2 : Sum  Inputs=|+-
  Transfer Fcn2 : TransferFcn  Denominator=[0.0075 0.5]
  q_3 : Outport
  i_3 : Outport  Port=2
  u_3 : Outport  Port=3
  q3pr : Outport  Port=4
  q3prpr : Outport  Port=5
  wires:
  Saturation1/1 -> u_3/1, Sum1/1
  Gain7/1 -> q3prpr/1
  Gain3/1 -> q3pr/1
  Gain2/1 -> Sum2/2
  Gain6/1 -> q_3/1
  P_3/1 -> Gain2/1
  Err_3/1 -> Saturation1/1
  Sum2/1 -> Gain4/1
  Gain4/1 -> Gain7/1, Integrator1/1
  Sum1/1 -> Transfer Fcn2/1
  Gain5/1 -> Sum1/2
  Integrator7/1 -> Gain6/1
  Integrator1/1 -> Integrator7/1, Gain3/1, Gain5/1
  Gain1/1 -> Sum2/1
  Transfer Fcn2/1 -> Gain1/1, i_3/1

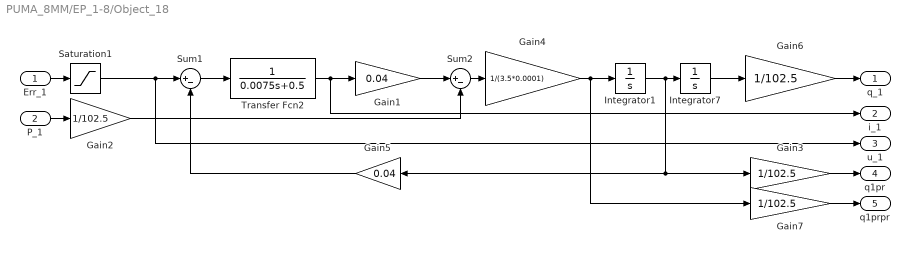
== system PUMA_8MM/EP_1-8/Object_18 ==
  Err_1 : Inport
  P_1 : Inport  Port=2
  Gain1 : Gain  Gain=0.04
  Gain{2..3,6..7} (4 alike) : Gain  Gain=1/102.5
  Gain4 : Gain  Gain=1/(3.5*0.0001)
  Gain5 : Gain  Gain=0.04
  Integrator1 : Integrator
  Integrator7 : Integrator  InitialCondition=0*102.5
  Saturation1 : Saturate  UpperLimit=30  LowerLimit=-30
  Sum1 : Sum  Inputs=|+-
  Sum2 : Sum  Inputs=|+-
  Transfer Fcn2 : TransferFcn  Denominator=[0.0075 0.5]
  q_1 : Outport
  i_1 : Outport  Port=2
  u_1 : Outport  Port=3
  q1pr : Outport  Port=4
  q1prpr : Outport  Port=5
  wires:
  Saturation1/1 -> u_1/1, Sum1/1
  Gain7/1 -> q1prpr/1
  Gain3/1 -> q1pr/1
  Gain2/1 -> Sum2/2
  Gain6/1 -> q_1/1
  P_1/1 -> Gain2/1
  Err_1/1 -> Saturation1/1
  Sum2/1 -> Gain4/1
  Gain4/1 -> Gain7/1, Integrator1/1
  Sum1/1 -> Transfer Fcn2/1
  Gain5/1 -> Sum1/2
  Integrator7/1 -> Gain6/1
  Integrator1/1 -> Integrator7/1, Gain3/1, Gain5/1
  Gain1/1 -> Sum2/1
  Transfer Fcn2/1 -> Gain1/1, i_1/1

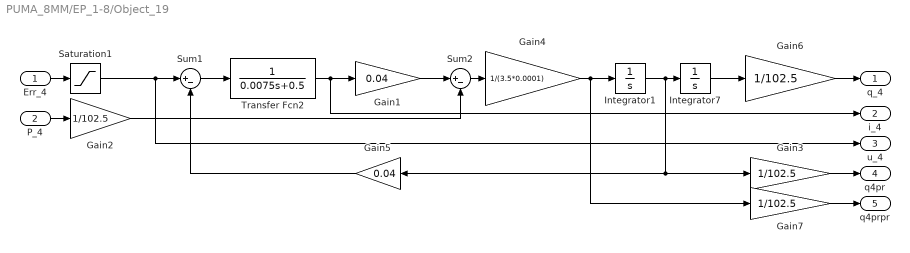
== system PUMA_8MM/EP_1-8/Object_19 ==
  Err_4 : Inport
  P_4 : Inport  Port=2
  Gain1 : Gain  Gain=0.04
  Gain{2..3,6..7} (4 alike) : Gain  Gain=1/102.5
  Gain4 : Gain  Gain=1/(3.5*0.0001)
  Gain5 : Gain  Gain=0.04
  Integrator1 : Integrator
  Integrator7 : Integrator  InitialCondition=1.57*102.5
  Saturation1 : Saturate  UpperLimit=30  LowerLimit=-30
  Sum1 : Sum  Inputs=|+-
  Sum2 : Sum  Inputs=|+-
  Transfer Fcn2 : TransferFcn  Denominator=[0.0075 0.5]
  q_4 : Outport
  i_4 : Outport  Port=2
  u_4 : Outport  Port=3
  q4pr : Outport  Port=4
  q4prpr : Outport  Port=5
  wires:
  Transfer Fcn2/1 -> i_4/1, Gain1/1
  Gain1/1 -> Sum2/1
  Integrator1/1 -> Gain5/1, Gain3/1, Integrator7/1
  Integrator7/1 -> Gain6/1
  Gain5/1 -> Sum1/2
  Sum1/1 -> Transfer Fcn2/1
  Gain4/1 -> Integrator1/1, Gain7/1
  Sum2/1 -> Gain4/1
  Err_4/1 -> Saturation1/1
  P_4/1 -> Gain2/1
  Gain6/1 -> q_4/1
  Gain2/1 -> Sum2/2
  Gain3/1 -> q4pr/1
  Gain7/1 -> q4prpr/1
  Saturation1/1 -> Sum1/1, u_4/1

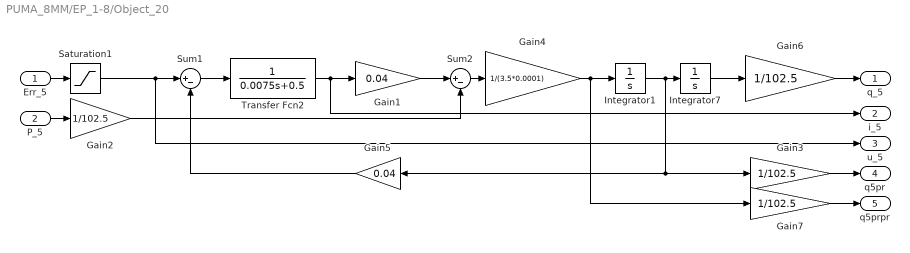
== system PUMA_8MM/EP_1-8/Object_20 ==
  Err_5 : Inport
  P_5 : Inport  Port=2
  Gain1 : Gain  Gain=0.04
  Gain{2..3,6..7} (4 alike) : Gain  Gain=1/102.5
  Gain4 : Gain  Gain=1/(3.5*0.0001)
  Gain5 : Gain  Gain=0.04
  Integrator1 : Integrator
  Integrator7 : Integrator  InitialCondition=0.667*102.5
  Saturation1 : Saturate  UpperLimit=30  LowerLimit=-30
  Sum1 : Sum  Inputs=|+-
  Sum2 : Sum  Inputs=|+-
  Transfer Fcn2 : TransferFcn  Denominator=[0.0075 0.5]
  q_5 : Outport
  i_5 : Outport  Port=2
  u_5 : Outport  Port=3
  q5pr : Outport  Port=4
  q5prpr : Outport  Port=5
  wires:
  Saturation1/1 -> u_5/1, Sum1/1
  Gain7/1 -> q5prpr/1
  Gain3/1 -> q5pr/1
  Gain2/1 -> Sum2/2
  Gain6/1 -> q_5/1
  P_5/1 -> Gain2/1
  Err_5/1 -> Saturation1/1
  Sum2/1 -> Gain4/1
  Gain4/1 -> Gain7/1, Integrator1/1
  Sum1/1 -> Transfer Fcn2/1
  Gain5/1 -> Sum1/2
  Integrator7/1 -> Gain6/1
  Integrator1/1 -> Integrator7/1, Gain3/1, Gain5/1
  Gain1/1 -> Sum2/1
  Transfer Fcn2/1 -> Gain1/1, i_5/1

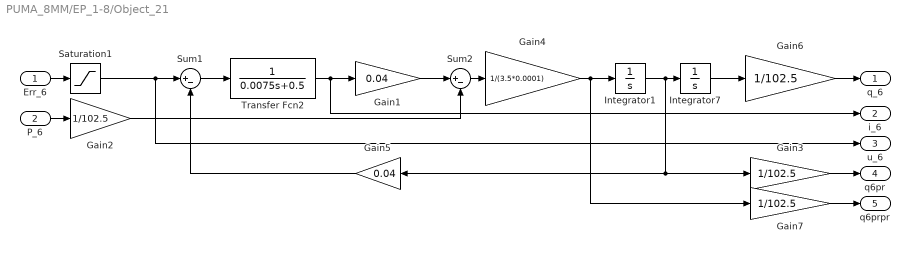
== system PUMA_8MM/EP_1-8/Object_21 ==
  Err_6 : Inport
  P_6 : Inport  Port=2
  Gain1 : Gain  Gain=0.04
  Gain{2..3,6..7} (4 alike) : Gain  Gain=1/102.5
  Gain4 : Gain  Gain=1/(3.5*0.0001)
  Gain5 : Gain  Gain=0.04
  Integrator1 : Integrator
  Integrator7 : Integrator  InitialCondition=-1.57*102.5
  Saturation1 : Saturate  UpperLimit=30  LowerLimit=-30
  Sum1 : Sum  Inputs=|+-
  Sum2 : Sum  Inputs=|+-
  Transfer Fcn2 : TransferFcn  Denominator=[0.0075 0.5]
  q_6 : Outport
  i_6 : Outport  Port=2
  u_6 : Outport  Port=3
  q6pr : Outport  Port=4
  q6prpr : Outport  Port=5
  wires:
  Transfer Fcn2/1 -> i_6/1, Gain1/1
  Gain1/1 -> Sum2/1
  Integrator1/1 -> Gain5/1, Gain3/1, Integrator7/1
  Integrator7/1 -> Gain6/1
  Gain5/1 -> Sum1/2
  Sum1/1 -> Transfer Fcn2/1
  Gain4/1 -> Integrator1/1, Gain7/1
  Sum2/1 -> Gain4/1
  Err_6/1 -> Saturation1/1
  P_6/1 -> Gain2/1
  Gain6/1 -> q_6/1
  Gain2/1 -> Sum2/2
  Gain3/1 -> q6pr/1
  Gain7/1 -> q6prpr/1
  Saturation1/1 -> Sum1/1, u_6/1

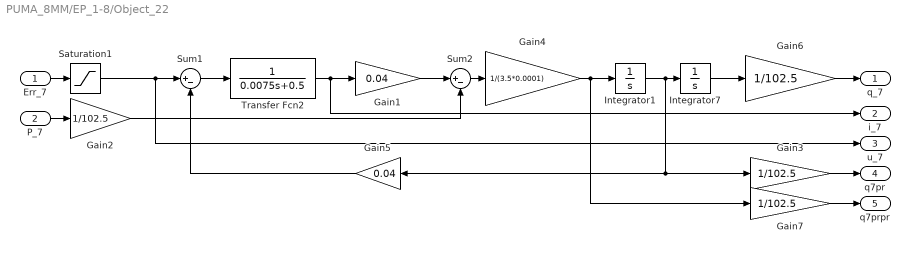
== system PUMA_8MM/EP_1-8/Object_22 ==
  Err_7 : Inport
  P_7 : Inport  Port=2
  Gain1 : Gain  Gain=0.04
  Gain{2..3,6..7} (4 alike) : Gain  Gain=1/102.5
  Gain4 : Gain  Gain=1/(3.5*0.0001)
  Gain5 : Gain  Gain=0.04
  Integrator1 : Integrator
  Integrator7 : Integrator  InitialCondition=-0.45*102.5
  Saturation1 : Saturate  UpperLimit=30  LowerLimit=-30
  Sum1 : Sum  Inputs=|+-
  Sum2 : Sum  Inputs=|+-
  Transfer Fcn2 : TransferFcn  Denominator=[0.0075 0.5]
  q_7 : Outport
  i_7 : Outport  Port=2
  u_7 : Outport  Port=3
  q7pr : Outport  Port=4
  q7prpr : Outport  Port=5
  wires:
  Saturation1/1 -> u_7/1, Sum1/1
  Gain7/1 -> q7prpr/1
  Gain3/1 -> q7pr/1
  Gain2/1 -> Sum2/2
  Gain6/1 -> q_7/1
  P_7/1 -> Gain2/1
  Err_7/1 -> Saturation1/1
  Sum2/1 -> Gain4/1
  Gain4/1 -> Gain7/1, Integrator1/1
  Sum1/1 -> Transfer Fcn2/1
  Gain5/1 -> Sum1/2
  Integrator7/1 -> Gain6/1
  Integrator1/1 -> Integrator7/1, Gain3/1, Gain5/1
  Gain1/1 -> Sum2/1
  Transfer Fcn2/1 -> Gain1/1, i_7/1

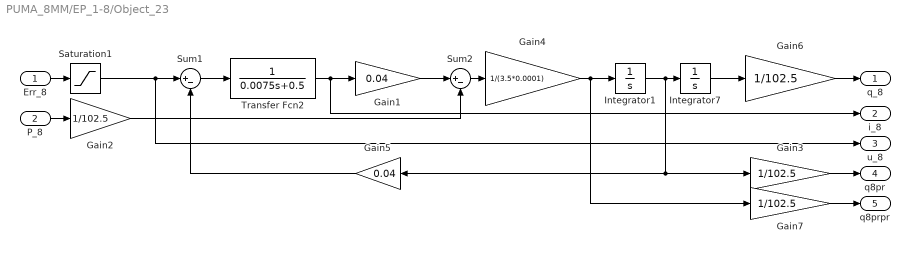
== system PUMA_8MM/EP_1-8/Object_23 ==
  Err_8 : Inport
  P_8 : Inport  Port=2
  Gain1 : Gain  Gain=0.04
  Gain{2..3,6..7} (4 alike) : Gain  Gain=1/102.5
  Gain4 : Gain  Gain=1/(3.5*0.0001)
  Gain5 : Gain  Gain=0.04
  Integrator1 : Integrator
  Integrator7 : Integrator  InitialCondition=0*102.5
  Saturation1 : Saturate  UpperLimit=30  LowerLimit=-30
  Sum1 : Sum  Inputs=|+-
  Sum2 : Sum  Inputs=|+-
  Transfer Fcn2 : TransferFcn  Denominator=[0.0075 0.5]
  q_8 : Outport
  i_8 : Outport  Port=2
  u_8 : Outport  Port=3
  q8pr : Outport  Port=4
  q8prpr : Outport  Port=5
  wires:
  Transfer Fcn2/1 -> i_8/1, Gain1/1
  Gain1/1 -> Sum2/1
  Integrator1/1 -> Gain5/1, Gain3/1, Integrator7/1
  Integrator7/1 -> Gain6/1
  Gain5/1 -> Sum1/2
  Sum1/1 -> Transfer Fcn2/1
  Gain4/1 -> Integrator1/1, Gain7/1
  Sum2/1 -> Gain4/1
  Err_8/1 -> Saturation1/1
  P_8/1 -> Gain2/1
  Gain6/1 -> q_8/1
  Gain2/1 -> Sum2/2
  Gain3/1 -> q8pr/1
  Gain7/1 -> q8prpr/1
  Saturation1/1 -> Sum1/1, u_8/1

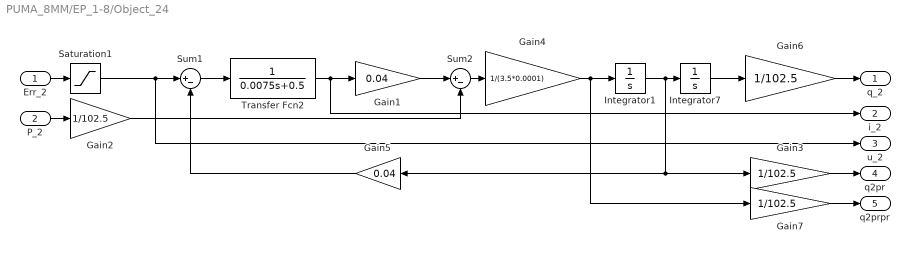
== system PUMA_8MM/EP_1-8/Object_24 ==
  Err_2 : Inport
  P_2 : Inport  Port=2
  Gain1 : Gain  Gain=0.04
  Gain{2..3,6..7} (4 alike) : Gain  Gain=1/102.5
  Gain4 : Gain  Gain=1/(3.5*0.0001)
  Gain5 : Gain  Gain=0.04
  Integrator1 : Integrator
  Integrator7 : Integrator  InitialCondition=0.667*102.5
  Saturation1 : Saturate  UpperLimit=30  LowerLimit=-30
  Sum1 : Sum  Inputs=|+-
  Sum2 : Sum  Inputs=|+-
  Transfer Fcn2 : TransferFcn  Denominator=[0.0075 0.5]
  q_2 : Outport
  i_2 : Outport  Port=2
  u_2 : Outport  Port=3
  q2pr : Outport  Port=4
  q2prpr : Outport  Port=5
  wires:
  Transfer Fcn2/1 -> i_2/1, Gain1/1
  Gain1/1 -> Sum2/1
  Integrator1/1 -> Gain5/1, Gain3/1, Integrator7/1
  Integrator7/1 -> Gain6/1
  Gain5/1 -> Sum1/2
  Sum1/1 -> Transfer Fcn2/1
  Gain4/1 -> Integrator1/1, Gain7/1
  Sum2/1 -> Gain4/1
  Err_2/1 -> Saturation1/1
  P_2/1 -> Gain2/1
  Gain6/1 -> q_2/1
  Gain2/1 -> Sum2/2
  Gain3/1 -> q2pr/1
  Gain7/1 -> q2prpr/1
  Saturation1/1 -> Sum1/1, u_2/1

== system PUMA_8MM/EP_1-8/Object_25 ==
  Err_3 : Inport
  P_3 : Inport  Port=2
  Gain1 : Gain  Gain=0.04
  Gain{2..3,6..7} (4 alike) : Gain  Gain=1/102.5
  Gain4 : Gain  Gain=1/(3.5*0.0001)
  Gain5 : Gain  Gain=0.04
  Integrator1 : Integrator
  Integrator7 : Integrator  InitialCondition=-1.5274*102.5
  Saturation1 : Saturate  UpperLimit=30  LowerLimit=-30
  Sum1 : Sum  Inputs=|+-
  Sum2 : Sum  Inputs=|+-
  Transfer Fcn2 : TransferFcn  Denominator=[0.0075 0.5]
  q_3 : Outport
  i_3 : Outport  Port=2
  u_3 : Outport  Port=3
  q3pr : Outport  Port=4
  q3prpr : Outport  Port=5
  wires:
  Saturation1/1 -> u_3/1, Sum1/1
  Gain7/1 -> q3prpr/1
  Gain3/1 -> q3pr/1
  Gain2/1 -> Sum2/2
  Gain6/1 -> q_3/1
  P_3/1 -> Gain2/1
  Err_3/1 -> Saturation1/1
  Sum2/1 -> Gain4/1
  Gain4/1 -> Gain7/1, Integrator1/1
  Sum1/1 -> Transfer Fcn2/1
  Gain5/1 -> Sum1/2
  Integrator7/1 -> Gain6/1
  Integrator1/1 -> Integrator7/1, Gain3/1, Gain5/1
  Gain1/1 -> Sum2/1
  Transfer Fcn2/1 -> Gain1/1, i_3/1

== system PUMA_8MM/EP_1-8/Object_26 ==
  Err_1 : Inport
  P_1 : Inport  Port=2
  Gain1 : Gain  Gain=0.04
  Gain{2..3,6..7} (4 alike) : Gain  Gain=1/102.5
  Gain4 : Gain  Gain=1/(3.5*0.0001)
  Gain5 : Gain  Gain=0.04
  Integrator1 : Integrator
  Integrator7 : Integrator  InitialCondition=0*102.5
  Saturation1 : Saturate  UpperLimit=30  LowerLimit=-30
  Sum1 : Sum  Inputs=|+-
  Sum2 : Sum  Inputs=|+-
  Transfer Fcn2 : TransferFcn  Denominator=[0.0075 0.5]
  q_1 : Outport
  i_1 : Outport  Port=2
  u_1 : Outport  Port=3
  q1pr : Outport  Port=4
  q1prpr : Outport  Port=5
  wires:
  Saturation1/1 -> u_1/1, Sum1/1
  Gain7/1 -> q1prpr/1
  Gain3/1 -> q1pr/1
  Gain2/1 -> Sum2/2
  Gain6/1 -> q_1/1
  P_1/1 -> Gain2/1
  Err_1/1 -> Saturation1/1
  Sum2/1 -> Gain4/1
  Gain4/1 -> Gain7/1, Integrator1/1
  Sum1/1 -> Transfer Fcn2/1
  Gain5/1 -> Sum1/2
  Integrator7/1 -> Gain6/1
  Integrator1/1 -> Integrator7/1, Gain3/1, Gain5/1
  Gain1/1 -> Sum2/1
  Transfer Fcn2/1 -> Gain1/1, i_1/1

== system PUMA_8MM/EP_1-8/Object_27 ==
  Err_4 : Inport
  P_4 : Inport  Port=2
  Gain1 : Gain  Gain=0.04
  Gain{2..3,6..7} (4 alike) : Gain  Gain=1/102.5
  Gain4 : Gain  Gain=1/(3.5*0.0001)
  Gain5 : Gain  Gain=0.04
  Integrator1 : Integrator
  Integrator7 : Integrator  InitialCondition=1.572*102.5
  Saturation1 : Saturate  UpperLimit=30  LowerLimit=-30
  Sum1 : Sum  Inputs=|+-
  Sum2 : Sum  Inputs=|+-
  Transfer Fcn2 : TransferFcn  Denominator=[0.0075 0.5]
  q_4 : Outport
  i_4 : Outport  Port=2
  u_4 : Outport  Port=3
  q4pr : Outport  Port=4
  q4prpr : Outport  Port=5
  wires:
  Transfer Fcn2/1 -> i_4/1, Gain1/1
  Gain1/1 -> Sum2/1
  Integrator1/1 -> Gain5/1, Gain3/1, Integrator7/1
  Integrator7/1 -> Gain6/1
  Gain5/1 -> Sum1/2
  Sum1/1 -> Transfer Fcn2/1
  Gain4/1 -> Integrator1/1, Gain7/1
  Sum2/1 -> Gain4/1
  Err_4/1 -> Saturation1/1
  P_4/1 -> Gain2/1
  Gain6/1 -> q_4/1
  Gain2/1 -> Sum2/2
  Gain3/1 -> q4pr/1
  Gain7/1 -> q4prpr/1
  Saturation1/1 -> Sum1/1, u_4/1

== system PUMA_8MM/EP_1-8/Object_28 ==
  Err_5 : Inport
  P_5 : Inport  Port=2
  Gain1 : Gain  Gain=0.04
  Gain{2..3,6..7} (4 alike) : Gain  Gain=1/102.5
  Gain4 : Gain  Gain=1/(3.5*0.0001)
  Gain5 : Gain  Gain=0.04
  Integrator1 : Integrator
  Integrator7 : Integrator  InitialCondition=0.9126*102.5
  Saturation1 : Saturate  UpperLimit=30  LowerLimit=-30
  Sum1 : Sum  Inputs=|+-
  Sum2 : Sum  Inputs=|+-
  Transfer Fcn2 : TransferFcn  Denominator=[0.0075 0.5]
  q_5 : Outport
  i_5 : Outport  Port=2
  u_5 : Outport  Port=3
  q5pr : Outport  Port=4
  q5prpr : Outport  Port=5
  wires:
  Saturation1/1 -> u_5/1, Sum1/1
  Gain7/1 -> q5prpr/1
  Gain3/1 -> q5pr/1
  Gain2/1 -> Sum2/2
  Gain6/1 -> q_5/1
  P_5/1 -> Gain2/1
  Err_5/1 -> Saturation1/1
  Sum2/1 -> Gain4/1
  Gain4/1 -> Gain7/1, Integrator1/1
  Sum1/1 -> Transfer Fcn2/1
  Gain5/1 -> Sum1/2
  Integrator7/1 -> Gain6/1
  Integrator1/1 -> Integrator7/1, Gain3/1, Gain5/1
  Gain1/1 -> Sum2/1
  Transfer Fcn2/1 -> Gain1/1, i_5/1

== system PUMA_8MM/EP_1-8/Object_29 ==
  Err_6 : Inport
  P_6 : Inport  Port=2
  Gain1 : Gain  Gain=0.04
  Gain{2..3,6..7} (4 alike) : Gain  Gain=1/102.5
  Gain4 : Gain  Gain=1/(3.5*0.0001)
  Gain5 : Gain  Gain=0.04
  Integrator1 : Integrator
  Integrator7 : Integrator  InitialCondition=-1.57*102.5
  Saturation1 : Saturate  UpperLimit=30  LowerLimit=-30
  Sum1 : Sum  Inputs=|+-
  Sum2 : Sum  Inputs=|+-
  Transfer Fcn2 : TransferFcn  Denominator=[0.0075 0.5]
  q_6 : Outport
  i_6 : Outport  Port=2
  u_6 : Outport  Port=3
  q6pr : Outport  Port=4
  q6prpr : Outport  Port=5
  wires:
  Transfer Fcn2/1 -> i_6/1, Gain1/1
  Gain1/1 -> Sum2/1
  Integrator1/1 -> Gain5/1, Gain3/1, Integrator7/1
  Integrator7/1 -> Gain6/1
  Gain5/1 -> Sum1/2
  Sum1/1 -> Transfer Fcn2/1
  Gain4/1 -> Integrator1/1, Gain7/1
  Sum2/1 -> Gain4/1
  Err_6/1 -> Saturation1/1
  P_6/1 -> Gain2/1
  Gain6/1 -> q_6/1
  Gain2/1 -> Sum2/2
  Gain3/1 -> q6pr/1
  Gain7/1 -> q6prpr/1
  Saturation1/1 -> Sum1/1, u_6/1

== system PUMA_8MM/EP_1-8/Object_30 ==
  Err_7 : Inport
  P_7 : Inport  Port=2
  Gain1 : Gain  Gain=0.04
  Gain{2..3,6..7} (4 alike) : Gain  Gain=1/102.5
  Gain4 : Gain  Gain=1/(3.5*0.0001)
  Gain5 : Gain  Gain=0.04
  Integrator1 : Integrator
  Integrator7 : Integrator  InitialCondition=-0.45*102.5
  Saturation1 : Saturate  UpperLimit=30  LowerLimit=-30
  Sum1 : Sum  Inputs=|+-
  Sum2 : Sum  Inputs=|+-
  Transfer Fcn2 : TransferFcn  Denominator=[0.0075 0.5]
  q_7 : Outport
  i_7 : Outport  Port=2
  u_7 : Outport  Port=3
  q7pr : Outport  Port=4
  q7prpr : Outport  Port=5
  wires:
  Saturation1/1 -> u_7/1, Sum1/1
  Gain7/1 -> q7prpr/1
  Gain3/1 -> q7pr/1
  Gain2/1 -> Sum2/2
  Gain6/1 -> q_7/1
  P_7/1 -> Gain2/1
  Err_7/1 -> Saturation1/1
  Sum2/1 -> Gain4/1
  Gain4/1 -> Gain7/1, Integrator1/1
  Sum1/1 -> Transfer Fcn2/1
  Gain5/1 -> Sum1/2
  Integrator7/1 -> Gain6/1
  Integrator1/1 -> Integrator7/1, Gain3/1, Gain5/1
  Gain1/1 -> Sum2/1
  Transfer Fcn2/1 -> Gain1/1, i_7/1

== system PUMA_8MM/EP_1-8/Object_31 ==
  Err_8 : Inport
  P_8 : Inport  Port=2
  Gain1 : Gain  Gain=0.04
  Gain{2..3,6..7} (4 alike) : Gain  Gain=1/102.5
  Gain4 : Gain  Gain=1/(3.5*0.0001)
  Gain5 : Gain  Gain=0.04
  Integrator1 : Integrator
  Integrator7 : Integrator  InitialCondition=0*102.5
  Saturation1 : Saturate  UpperLimit=30  LowerLimit=-30
  Sum1 : Sum  Inputs=|+-
  Sum2 : Sum  Inputs=|+-
  Transfer Fcn2 : TransferFcn  Denominator=[0.0075 0.5]
  q_8 : Outport
  i_8 : Outport  Port=2
  u_8 : Outport  Port=3
  q8pr : Outport  Port=4
  q8prpr : Outport  Port=5
  wires:
  Transfer Fcn2/1 -> i_8/1, Gain1/1
  Gain1/1 -> Sum2/1
  Integrator1/1 -> Gain5/1, Gain3/1, Integrator7/1
  Integrator7/1 -> Gain6/1
  Gain5/1 -> Sum1/2
  Sum1/1 -> Transfer Fcn2/1
  Gain4/1 -> Integrator1/1, Gain7/1
  Sum2/1 -> Gain4/1
  Err_8/1 -> Saturation1/1
  P_8/1 -> Gain2/1
  Gain6/1 -> q_8/1
  Gain2/1 -> Sum2/2
  Gain3/1 -> q8pr/1
  Gain7/1 -> q8prpr/1
  Saturation1/1 -> Sum1/1, u_8/1

== system PUMA_8MM/EP_1-8/Object_32 ==
  Err_2 : Inport
  P_2 : Inport  Port=2
  Gain1 : Gain  Gain=0.04
  Gain{2..3,6..7} (4 alike) : Gain  Gain=1/102.5
  Gain4 : Gain  Gain=1/(3.5*0.0001)
  Gain5 : Gain  Gain=0.04
  Integrator1 : Integrator
  Integrator7 : Integrator  InitialCondition=0.6147*102.5
  Saturation1 : Saturate  UpperLimit=30  LowerLimit=-30
  Sum1 : Sum  Inputs=|+-
  Sum2 : Sum  Inputs=|+-
  Transfer Fcn2 : TransferFcn  Denominator=[0.0075 0.5]
  q_2 : Outport
  i_2 : Outport  Port=2
  u_2 : Outport  Port=3
  q2pr : Outport  Port=4
  q2prpr : Outport  Port=5
  wires:
  Transfer Fcn2/1 -> i_2/1, Gain1/1
  Gain1/1 -> Sum2/1
  Integrator1/1 -> Gain5/1, Gain3/1, Integrator7/1
  Integrator7/1 -> Gain6/1
  Gain5/1 -> Sum1/2
  Sum1/1 -> Transfer Fcn2/1
  Gain4/1 -> Integrator1/1, Gain7/1
  Sum2/1 -> Gain4/1
  Err_2/1 -> Saturation1/1
  P_2/1 -> Gain2/1
  Gain6/1 -> q_2/1
  Gain2/1 -> Sum2/2
  Gain3/1 -> q2pr/1
  Gain7/1 -> q2prpr/1
  Saturation1/1 -> Sum1/1, u_2/1

== system PUMA_8MM/EP_1-8/Object_9 ==
  Err_2 : Inport
  P_2 : Inport  Port=2
  Gain1 : Gain  Gain=0.04
  Gain{2..3,6..7} (4 alike) : Gain  Gain=1/102.5
  Gain4 : Gain  Gain=1/(3.5*0.0001)
  Gain5 : Gain  Gain=0.04
  Integrator1 : Integrator
  Integrator7 : Integrator  InitialCondition=0.7894*102.5
  Sum1 : Sum  Inputs=|+-
  Sum2 : Sum  Inputs=|+-
  Transfer Fcn2 : TransferFcn  Denominator=[0.0075 0.5]
  q_2 : Outport
  i_2 : Outport  Port=2
  u_2 : Outport  Port=3
  q2pr : Outport  Port=4
  q2prpr : Outport  Port=5
  wires:
  Transfer Fcn2/1 -> i_2/1, Gain1/1
  Gain1/1 -> Sum2/1
  Integrator1/1 -> Gain5/1, Gain3/1, Integrator7/1
  Integrator7/1 -> Gain6/1
  Gain5/1 -> Sum1/2
  Sum1/1 -> Transfer Fcn2/1
  Gain4/1 -> Integrator1/1, Gain7/1
  Sum2/1 -> Gain4/1
  Err_2/1 -> Sum1/1, u_2/1
  P_2/1 -> Gain2/1
  Gain6/1 -> q_2/1
  Gain2/1 -> Sum2/2
  Gain3/1 -> q2pr/1
  Gain7/1 -> q2prpr/1

== system PUMA_8MM/EP_1-8/PID_zveno_1 ==
  in_2 : Inport
  Gain3 : Gain  Gain=5
  PID_1 : Subsystem
  on/off_2 : ManualSwitch
  out_PID_2 : Outport
  wires:
  on/off_2/1 -> Gain3/1
  in_2/1 -> PID_1/1(in), on/off_2/2
  PID_1/1(out) -> on/off_2/1
  Gain3/1 -> out_PID_2/1

== system PUMA_8MM/EP_1-8/PID_zveno_2 ==
  in_3 : Inport
  Gain3 : Gain  Gain=5
  PID_1 : Subsystem
  on/off_3 : ManualSwitch
  out_PID_3 : Outport
  wires:
  Gain3/1 -> out_PID_3/1
  PID_1/1(out) -> on/off_3/1
  in_3/1 -> on/off_3/2, PID_1/1(in)
  on/off_3/1 -> Gain3/1

== system PUMA_8MM/EP_1-8/PID_zveno_3 ==
  in_1 : Inport
  Gain3 : Gain  Gain=5
  PID_1 : Subsystem
  on/off_1 : ManualSwitch
  out_PID_1 : Outport
  wires:
  Gain3/1 -> out_PID_1/1
  PID_1/1(out) -> on/off_1/1
  in_1/1 -> on/off_1/2, PID_1/1(in)
  on/off_1/1 -> Gain3/1

== system PUMA_8MM/EP_1-8/PID_zveno_4 ==
  in_4 : Inport
  Gain3 : Gain  Gain=5
  PID_1 : Subsystem
  on/off_4 : ManualSwitch
  out_PID_4 : Outport
  wires:
  on/off_4/1 -> Gain3/1
  in_4/1 -> PID_1/1(in), on/off_4/2
  PID_1/1(out) -> on/off_4/1
  Gain3/1 -> out_PID_4/1

== system PUMA_8MM/EP_1-8/PID_zveno_5 ==
  in_5 : Inport
  Gain3 : Gain  Gain=5
  PID_1 : Subsystem
  on/off_5 : ManualSwitch
  out_PID_5 : Outport
  wires:
  Gain3/1 -> out_PID_5/1
  PID_1/1(out) -> on/off_5/1
  in_5/1 -> on/off_5/2, PID_1/1(in)
  on/off_5/1 -> Gain3/1

== system PUMA_8MM/EP_1-8/PID_zveno_6 ==
  in_6 : Inport
  Gain3 : Gain  Gain=5
  PID_1 : Subsystem
  on/off_6 : ManualSwitch
  out_PID_6 : Outport
  wires:
  on/off_6/1 -> Gain3/1
  in_6/1 -> PID_1/1(in), on/off_6/2
  PID_1/1(out) -> on/off_6/1
  Gain3/1 -> out_PID_6/1

== system PUMA_8MM/EP_1-8/PID_zveno_7 ==
  in_7 : Inport
  Gain3 : Gain  Gain=5
  PID_1 : Subsystem
  on/off_7 : ManualSwitch
  out_PID_7 : Outport
  wires:
  Gain3/1 -> out_PID_7/1
  PID_1/1(out) -> on/off_7/1
  in_7/1 -> on/off_7/2, PID_1/1(in)
  on/off_7/1 -> Gain3/1

== system PUMA_8MM/EP_1-8/PID_zveno_8 ==
  in_8 : Inport
  Gain3 : Gain  Gain=5
  PID_1 : Subsystem
  on/off_8 : ManualSwitch
  out_PID_8 : Outport
  wires:
  on/off_8/1 -> Gain3/1
  in_8/1 -> PID_1/1(in), on/off_8/2
  PID_1/1(out) -> on/off_8/1
  Gain3/1 -> out_PID_8/1

== system PUMA_8MM/EP_1-8/PID_zveno_1/PID_1 ==
  in : Inport
  Derivative : Derivative
  Gain : Gain  Gain=942.1595
  Gain1 : Gain  Gain=28.7683
  Gain2 : Gain  Gain=813.1589
  Gain3 : Gain
  Integrator : Integrator
  Sum : Sum  Inputs=+++
  out : Outport
  wires:
  Sum/1 -> Gain3/1
  in/1 -> Gain2/1, Integrator/1, Derivative/1
  Gain/1 -> Sum/1
  Gain1/1 -> Sum/2
  Gain2/1 -> Sum/3
  Derivative/1 -> Gain1/1
  Integrator/1 -> Gain/1
  Gain3/1 -> out/1

== system PUMA_8MM/EP_1-8/PID_zveno_2/PID_1 ==
  in : Inport
  Derivative : Derivative
  Gain : Gain  Gain=942.1595
  Gain1 : Gain  Gain=28.7683
  Gain2 : Gain  Gain=813.1589
  Gain3 : Gain
  Integrator : Integrator
  Sum : Sum  Inputs=+++
  out : Outport
  wires:
  Gain3/1 -> out/1
  Integrator/1 -> Gain/1
  Derivative/1 -> Gain1/1
  Gain2/1 -> Sum/3
  Gain1/1 -> Sum/2
  Gain/1 -> Sum/1
  in/1 -> Derivative/1, Integrator/1, Gain2/1
  Sum/1 -> Gain3/1

== system PUMA_8MM/EP_1-8/PID_zveno_3/PID_1 ==
  in : Inport
  Derivative : Derivative
  Gain : Gain  Gain=942.1595
  Gain1 : Gain  Gain=28.7683
  Gain2 : Gain  Gain=813.1589
  Gain3 : Gain
  Integrator : Integrator
  Sum : Sum  Inputs=+++
  out : Outport
  wires:
  Gain3/1 -> out/1
  Integrator/1 -> Gain/1
  Derivative/1 -> Gain1/1
  Gain2/1 -> Sum/3
  Gain1/1 -> Sum/2
  Gain/1 -> Sum/1
  in/1 -> Derivative/1, Integrator/1, Gain2/1
  Sum/1 -> Gain3/1

== system PUMA_8MM/EP_1-8/PID_zveno_4/PID_1 ==
  in : Inport
  Derivative : Derivative
  Gain : Gain  Gain=942.1595
  Gain1 : Gain  Gain=28.7683
  Gain2 : Gain  Gain=813.1589
  Gain3 : Gain
  Integrator : Integrator
  Sum : Sum  Inputs=+++
  out : Outport
  wires:
  Sum/1 -> Gain3/1
  in/1 -> Gain2/1, Integrator/1, Derivative/1
  Gain/1 -> Sum/1
  Gain1/1 -> Sum/2
  Gain2/1 -> Sum/3
  Derivative/1 -> Gain1/1
  Integrator/1 -> Gain/1
  Gain3/1 -> out/1

== system PUMA_8MM/EP_1-8/PID_zveno_5/PID_1 ==
  in : Inport
  Derivative : Derivative
  Gain : Gain  Gain=942.1595
  Gain1 : Gain  Gain=28.7683
  Gain2 : Gain  Gain=813.1589
  Gain3 : Gain
  Integrator : Integrator
  Sum : Sum  Inputs=+++
  out : Outport
  wires:
  Gain3/1 -> out/1
  Integrator/1 -> Gain/1
  Derivative/1 -> Gain1/1
  Gain2/1 -> Sum/3
  Gain1/1 -> Sum/2
  Gain/1 -> Sum/1
  in/1 -> Derivative/1, Integrator/1, Gain2/1
  Sum/1 -> Gain3/1

== system PUMA_8MM/EP_1-8/PID_zveno_6/PID_1 ==
  in : Inport
  Derivative : Derivative
  Gain : Gain  Gain=942.1595
  Gain1 : Gain  Gain=28.7683
  Gain2 : Gain  Gain=813.1589
  Gain3 : Gain
  Integrator : Integrator
  Sum : Sum  Inputs=+++
  out : Outport
  wires:
  Sum/1 -> Gain3/1
  in/1 -> Gain2/1, Integrator/1, Derivative/1
  Gain/1 -> Sum/1
  Gain1/1 -> Sum/2
  Gain2/1 -> Sum/3
  Derivative/1 -> Gain1/1
  Integrator/1 -> Gain/1
  Gain3/1 -> out/1

== system PUMA_8MM/EP_1-8/PID_zveno_7/PID_1 ==
  in : Inport
  Derivative : Derivative
  Gain : Gain  Gain=942.1595
  Gain1 : Gain  Gain=28.7683
  Gain2 : Gain  Gain=813.1589
  Gain3 : Gain
  Integrator : Integrator
  Sum : Sum  Inputs=+++
  out : Outport
  wires:
  Gain3/1 -> out/1
  Integrator/1 -> Gain/1
  Derivative/1 -> Gain1/1
  Gain2/1 -> Sum/3
  Gain1/1 -> Sum/2
  Gain/1 -> Sum/1
  in/1 -> Derivative/1, Integrator/1, Gain2/1
  Sum/1 -> Gain3/1

== system PUMA_8MM/EP_1-8/PID_zveno_8/PID_1 ==
  in : Inport
  Derivative : Derivative
  Gain : Gain  Gain=942.1595
  Gain1 : Gain  Gain=28.7683
  Gain2 : Gain  Gain=813.1589
  Gain3 : Gain
  Integrator : Integrator
  Sum : Sum  Inputs=+++
  out : Outport
  wires:
  Sum/1 -> Gain3/1
  in/1 -> Gain2/1, Integrator/1, Derivative/1
  Gain/1 -> Sum/1
  Gain1/1 -> Sum/2
  Gain2/1 -> Sum/3
  Derivative/1 -> Gain1/1
  Integrator/1 -> Gain/1
  Gain3/1 -> out/1

== matlab function OZK ==
  data: rx input double; ry input double; rz input double; q1 output double; q2 output double; q3 output double; q4 output double; q5 output double; q6 output double; ax input double; ay input double; az input double; bx input double; by input double; bz input double
function [q1,q2,q3,q4,q5,q6] = fcn(rx,ry,rz,ax,ay,az,bx,by,bz)

    % ОЗК для 6ти степенного ММ_ 
    pi = 3.14159265358979;
    % длины звеньев_
    L1 = 0.4;
    L2 = 0.7;
    L3 = 0.7;
    L4 = 0.1;
    
    % ограничения по степеням подвижности_ 
    % -pi/2 < qi < pi/2
    % -pi/2 < fi < pi/2, где fi=q2+q3
    
    Rx = rx-ax*L4;
    Ry = ry-ay*L4;
    Rz = rz-az*L4;
 
  if (Ry==0) Ry = 0.0000001; end;  
  q1 = -atan(Rx/Ry);
  
    f1 = (Rz-L1)/L3;
    f2 = -L2/L3;
    f3 = Ry/(L3*cos(q1));
    
    g1 = 2*f1*f2;
    g2 = 2*f2*f3;
    g3 = 1-f1*f1-f2*f2-f3*f3;
           
  q2 = asin(g3/sqrt(g1*g1+g2*g2)) - atan(f3/f1); 
    if (q2<-pi/2) q2 = q2+pi; end; % 
  q3 = asin(f1+f2*sin(q2)) - q2;   
  
    fi  = q2+q3;  
    sfi = sin(fi);
    cfi = cos(fi);
    if (ay==0) ay = 0.0000001; end;  
    alfa = -q1 - atan(ax/ay); 
    if (abs(alfa)<0.0000001) alfa = 0; end;

  if (alfa >= 0) q5 =  acos(-ax*sin(q1)*cfi + ay*cos(q1)*cfi + az*sfi); 
  else           q5 = -acos(-ax*sin(q1)*cfi + ay*cos(q1)*cfi + az*sfi);
  end;                                                                 
  
    k = az - sfi*cos(q5);

  if (q5==0) q5 = 0.0000001; end;
  q4 = acos((-ax*cos(q1)-ay*sin(q1))/sin(q5));
  if (k  < 0) q4 = -q4; end; 
  if (q5 < 0) q4 = -q4; end; 
    
    gammax =  bz*(sin(q1)*sin(q4) - cos(q1)*sfi*cos(q4)) - by*cfi*cos(q4);
    gammay = -bz*(cos(q1)*sin(q4) + sin(q1)*sfi*cos(q4)) + bx*cfi*cos(q4);
    
    betta = gammax*ax + gammay*ay;
    
  q6 = acos(  bx*(cos(q1)*sin(q4)+sin(q1)*sfi*cos(q4))  +  by*(sin(q1)*sin(q4)-cos(q1)*sfi*cos(q4))  +  bz*(cfi*cos(q4))  );
  if (betta<0)  q6 = -q6; end; 
  
  if (q1<-pi/2) q1 = -pi/2; end; 
  if (q1> pi/2) q1 =  pi/2; end;
  if (q2<-pi/2) q2 = -pi/2; end; 
  if (q2> pi/2) q2 =  pi/2; end;
  if (q3<-pi/2) q3 = -pi/2; end; 
  if (q3> pi/2) q3 =  pi/2; end;
  if (q4<-pi/2) q4 = -pi/2; end; 
  if (q4> pi/2) q4 =  pi/2; end;
  if (q5<-pi/2) q5 = -pi/2; end; 
  if (q5> pi/2) q5 =  pi/2; end;
  if (q6<-pi/2) q6 = -pi/2; end; 
  if (q6> pi/2) q6 =  pi/2; end;
  
end

== matlab function Corect2 ==
  data: x input double; rx output double; y input double; z input double; q7 input double; q8 input double; ry output double; rz output double; del1 output double; del2 output double
function [rx,ry,rz,del1,del2]  = fcn(x,y,z,q7,q8)
 
  rx = x - q7;
  ry = y - q8;
  rz = z     ;
  
  del1 = 0;
  del2 = 0;
           
end

== matlab function E_calc ==
  data: xr input double; E output double; yr input double; zr input double; xi input double; yi input double; zi input double
function E = fcn(xr,yr,zr,xi,yi,zi)

% xr and yr = x_real  and y_real
% xi and yi = x_ideal and y_idel
% zi and zi = z_ideal and z_idel

  E = sqrt(   (xi-xr)^2 + (yi-yr)^2 + (zi-zr)^2  );
           
end

== matlab function BFq7_alfa ==
  data: ax input double; ay input double; az input double; x input double; y input double; q7 output double
function q7  = fcn(ax,ay,az,x,y)
  
  L4   = 0.1;
  q8   = 0;
  alfa = 0.01;

  % alfa = var_
  %q7 = (ay*L4-y+q8)*tan( alfa + atan(ax/ay) ) - ax*L4 + x;
  q7 = x - ax*L4 - (y-ay*L4-q8)*tan( alfa + atan(ax/ay) );
  
  % alfa = const = 0_
  %q7 = x - ax/ay*y; 
  
end
